simulink model "MMS_ESC_K_B_self_driving"  (R2019b)
settings: Solver=ode45  StartTime=par.sym.TStart  StopTime=par.sym.TStop  MaxStep=par.sym.max_dt  RelTol=1e-3  EnableMultiTasking=on
undefined symbols (not defined in the file): b, B_0, BASE, eta_B, eta_K, k, K_0, lambda_B, lambda_K, m, m1_B0, m1_K0, m2_B0, m2_K0, N_delay, par, Q1_B0, Q1_K0, Q2_B0, Q2_K0, sigma, T_tran, w_L, w_wav
libraries: simulink x1
settings Model: Creator=Vitù  LastModifiedBy=User
settings DataIOCC: SaveFormat=Array  SaveOutput=off  SignalLogging=off  DSMLogging=off  ReturnWorkspaceOutputs=off  TimeSaveName=TIME  OutputSaveName=Yout  OutputOption=SpecifiedOutputTimes  OutputTimes=[par.sym.TStart:par.sym.Outputdt:par.sym.TStop]
settings OptimizationCC: ExpressionDepthLimit=2147483647  LifeSpan=inf
settings DebuggingCC: UnderspecifiedInitializationDetection=Classic  MergeDetectMultiDrivingBlocksExec=none  SolverPrmCheckMsg=warning  AllowSymbolicDim=off  StateNameClashWarn=warning  SFUnexpectedBacktrackingDiag=warning  SFNoUnconditionalDefaultTransitionDiag=warning  SFExecutionAtInitializationDiag=none  ArithmeticOperatorsInVariantConditions=warning
settings HardwareCC: ProdBitPerPointer=32  ProdBitPerSizeT=32  ProdBitPerPtrDiffT=32  ProdLargestAtomicFloat=None  ProdIntDivRoundTo=Undefined  ProdEndianess=Unspecified  ProdWordSize=32  ProdHWDeviceType=32-bit Generic
settings ModelReferenceCC: PropagateSignalLabelsOutOfModel=off
settings SFSimCC: SimUseLocalCustomCode=off  CustomCodeUndefinedFunction=UseInterfaceOnly
settings RTWCC: RTWUseLocalCustomCode=off
settings CodeAppCC: StateflowObjectComments=on
settings GRTTargetCC: TargetLangStandard=C89/C90 (ANSI)  GeneratePreprocessorConditionals=Disable all
settings ConfigComp: CovMetricSettings=dw  CovHtmlReporting=on  CovSaveCumulativeToWorkspaceVar=on  CovSaveSingleToWorkspaceVar=on  CovExternalEMLEnable=off  CovSFcnEnable=off
settings SimscapeCC: SimscapeNormalizeSystem=off
settings ConfigurationSet: Description=SimMechanics 2G

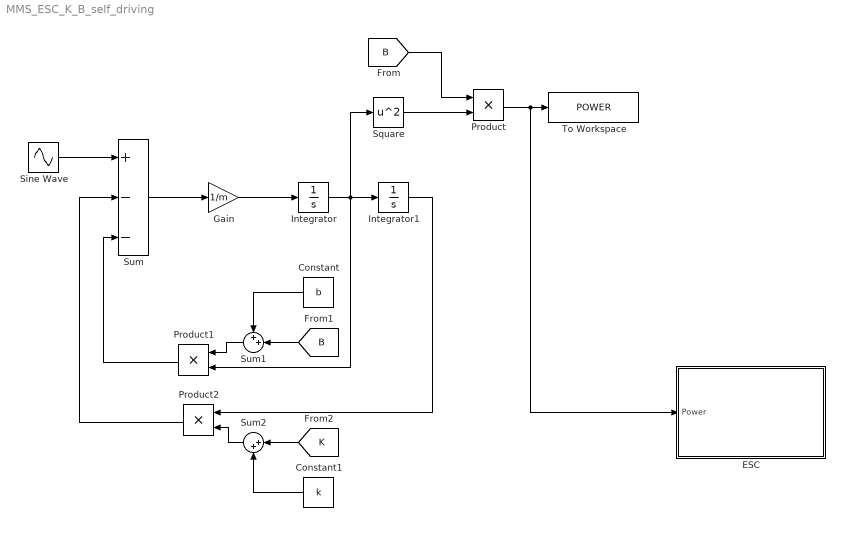
== system MMS_ESC_K_B_self_driving ==
  Constant : Constant  Value=b
  Constant1 : Constant  Value=k
  ESC : Subsystem
  Gain : Gain  Gain=1/m
  Integrator : Integrator
  Integrator1 : Integrator
  Product : Product
  Product1 : Product
  Product2 : Product
  Sine Wave : Sin  Amplitude=par.H  Frequency=w_wav  SampleTime=0
  Square : Math  Operator=square  SignedPower=off  SaturateOnIntegerOverflow=on
  Sum : Sum  Inputs=+--
  Sum1 : Sum  Inputs=++|
  Sum2 : Sum  Inputs=|++
  To Workspace : ToWorkspace  VariableName=POWER  SampleTime=-1
  wires:
  Integrator1/1 -> Product2/1
  Product/1 -> ESC/1(Power), To Workspace/1
  Product1/1 -> Sum/3
  Gain/1 -> Integrator/1
  Square/1 -> Product/2
  Sum/1 -> Gain/1
  Integrator/1 -> Product1/2, Square/1, Integrator1/1
  Product2/1 -> Sum/2
  Sine Wave/1 -> Sum/1
  [B] -> Product/1
  [B] -> Sum1/2
  Sum1/1 -> Product1/1
  Constant/1 -> Sum1/1
  [K] -> Sum2/1
  Sum2/1 -> Product2/2
  Constant1/1 -> Sum2/2

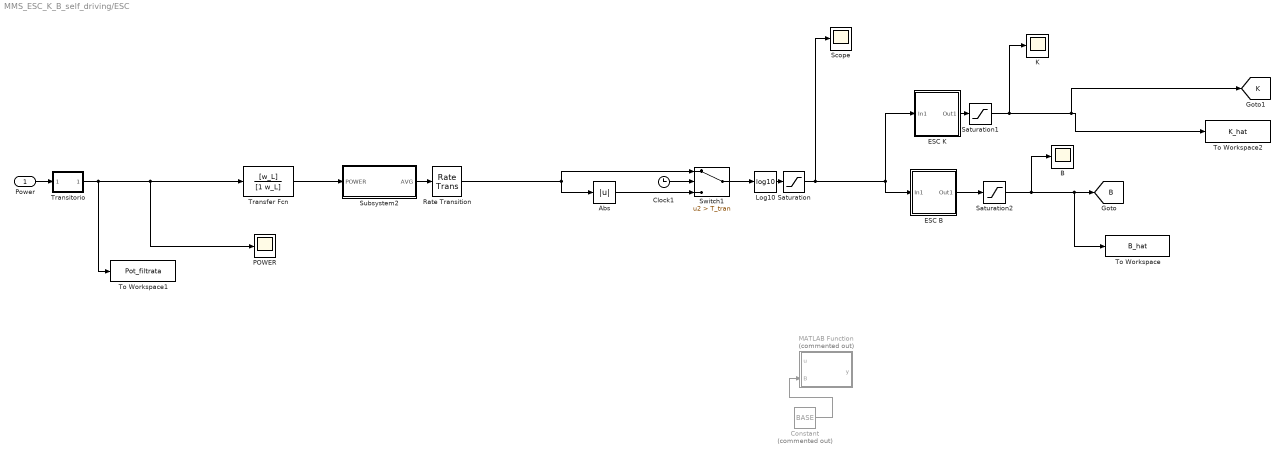
== system MMS_ESC_K_B_self_driving/ESC ==
  Power : Inport
  Abs : Abs
  B : Scope
  Clock1 : Clock
  Constant : Constant  Commented=on  Value=BASE
  ESC B : Subsystem
  ESC K : Subsystem
  K : Scope
  Log10 : Math  Operator=log10  SignedPower=off  SaturateOnIntegerOverflow=on
  MATLAB Function : MATLAB Function  Commented=on  TreatAsAtomicUnit=on
  POWER : Scope
  Rate Transition : RateTransition
  Saturation : Saturate  UpperLimit=inf  LowerLimit=-20
  Saturation1 : Saturate  UpperLimit=inf  LowerLimit=-k
  Saturation2 : Saturate  UpperLimit=inf  LowerLimit=-b
  Scope : Scope
  Subsystem2 : Subsystem
  Switch1 : Switch  Criteria=u2 > Threshold  Threshold=T_tran
  To Workspace : ToWorkspace  VariableName=B_hat  SampleTime=-1
  To Workspace1 : ToWorkspace  VariableName=Pot_filtrata  SampleTime=-1
  To Workspace2 : ToWorkspace  VariableName=K_hat  SampleTime=-1
  Transfer Fcn : TransferFcn  Numerator=[w_L]  Denominator=[1 w_L]
  Transitorio : Subsystem
  tag scope: B=global, K=global
  wires:
  Power/1 -> Transitorio/1(In1)
  ESC B/1(Out1) -> Saturation2/1
  ESC K/1(Out1) -> Saturation1/1
  Subsystem2/1(AVG) -> Rate Transition/1
  Constant/1 -> MATLAB Function/2(B)
  Log10/1 -> Saturation/1
  Transitorio/1(Out1) -> Transfer Fcn/1, POWER/1, To Workspace1/1
  Saturation/1 -> ESC B/1(In1), ESC K/1(In1), Scope/1
  Transfer Fcn/1 -> Subsystem2/1(POWER)
  Saturation1/1 -> K/1, [K], To Workspace2/1
  Saturation2/1 -> B/1, [B], To Workspace/1
  Switch1/1 -> Log10/1
  Rate Transition/1 -> Switch1/1, Abs/1
  Clock1/1 -> Switch1/2
  Abs/1 -> Switch1/3

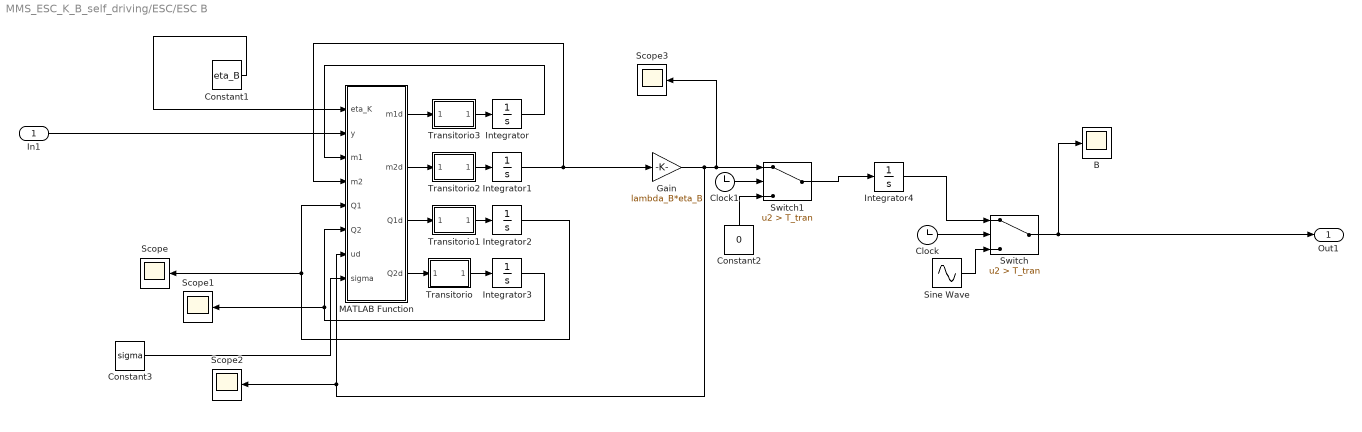
== system MMS_ESC_K_B_self_driving/ESC/ESC B ==
  In1 : Inport
  B : Scope
  Clock : Clock
  Clock1 : Clock
  Constant1 : Constant  Value=eta_B
  Constant2 : Constant  Value=0
  Constant3 : Constant  Value=sigma
  Gain : Gain  Gain=lambda_B*eta_B
  Integrator : Integrator  InitialCondition=m1_B0
  Integrator1 : Integrator  InitialCondition=m2_B0
  Integrator2 : Integrator  InitialCondition=Q1_B0
  Integrator3 : Integrator  InitialCondition=Q2_B0
  Integrator4 : Integrator  InitialCondition=B_0
  MATLAB Function : MATLAB Function  TreatAsAtomicUnit=on
  Scope{,1..3} (4 alike) : Scope
  Sine Wave : Sin  Bias=B_0  SampleTime=0
  Switch : Switch  Criteria=u2 > Threshold  Threshold=T_tran
  Switch1 : Switch  Criteria=u2 > Threshold  Threshold=T_tran
  Transitorio : Subsystem
  Transitorio1 : Subsystem
  Transitorio2 : Subsystem
  Transitorio3 : Subsystem
  Out1 : Outport
  wires:
  Switch/1 -> Out1/1, B/1
  Integrator2/1 -> MATLAB Function/5(Q1), Scope/1
  Constant2/1 -> Switch1/3
  Gain/1 -> Scope3/1, Switch1/1, MATLAB Function/7(ud), Scope2/1
  Integrator1/1 -> Gain/1, MATLAB Function/4(m2)
  MATLAB Function/4(Q2d) -> Transitorio/1(In1)
  Integrator/1 -> MATLAB Function/3(m1)
  In1/1 -> MATLAB Function/2(y)
  Switch1/1 -> Integrator4/1
  MATLAB Function/1(m1d) -> Transitorio3/1(In1)
  Integrator3/1 -> MATLAB Function/6(Q2), Scope1/1
  Sine Wave/1 -> Switch/3
  MATLAB Function/2(m2d) -> Transitorio2/1(In1)
  Clock1/1 -> Switch1/2
  MATLAB Function/3(Q1d) -> Transitorio1/1(In1)
  Constant1/1 -> MATLAB Function/1(eta_K)
  Constant3/1 -> MATLAB Function/8(sigma)
  Integrator4/1 -> Switch/1
  Clock/1 -> Switch/2
  Transitorio/1(Out1) -> Integrator3/1
  Transitorio1/1(Out1) -> Integrator2/1
  Transitorio2/1(Out1) -> Integrator1/1
  Transitorio3/1(Out1) -> Integrator/1

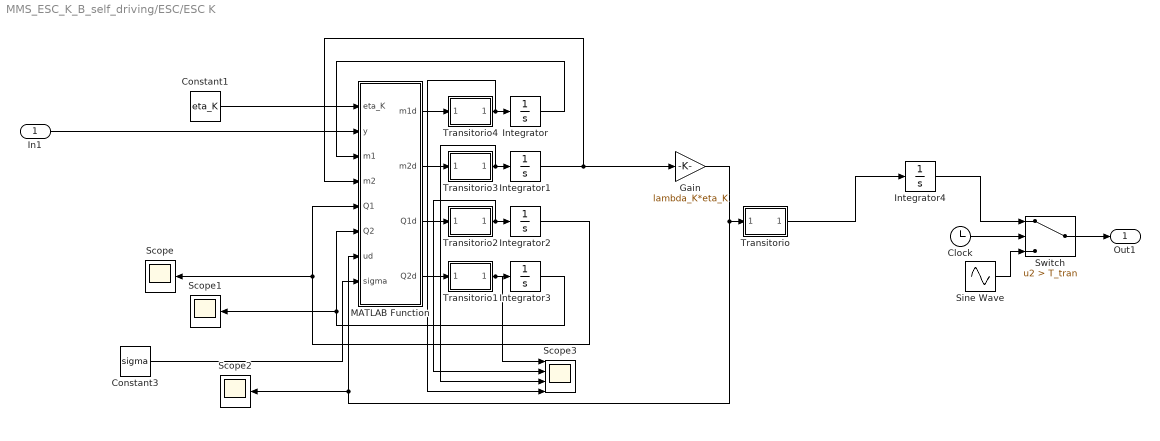
== system MMS_ESC_K_B_self_driving/ESC/ESC K ==
  In1 : Inport
  Clock : Clock
  Constant1 : Constant  Value=eta_K
  Constant3 : Constant  Value=sigma
  Gain : Gain  Gain=lambda_K*eta_K
  Integrator : Integrator  InitialCondition=m1_K0
  Integrator1 : Integrator  InitialCondition=m2_K0
  Integrator2 : Integrator  InitialCondition=Q1_K0
  Integrator3 : Integrator  InitialCondition=Q2_K0
  Integrator4 : Integrator  InitialCondition=K_0
  MATLAB Function : MATLAB Function  TreatAsAtomicUnit=on
  Scope : Scope
  Scope1 : Scope
  Scope2 : Scope
  Scope3 : Scope  NumInputPorts=4
  Sine Wave : Sin  Bias=K_0  SampleTime=0
  Switch : Switch  Criteria=u2 > Threshold  Threshold=T_tran
  Transitorio : Subsystem
  Transitorio1 : Subsystem
  Transitorio2 : Subsystem
  Transitorio3 : Subsystem
  Transitorio4 : Subsystem
  Out1 : Outport
  wires:
  Sine Wave/1 -> Switch/3
  Gain/1 -> Transitorio/1(In1), MATLAB Function/7(ud), Scope2/1
  Constant1/1 -> MATLAB Function/1(eta_K)
  Integrator1/1 -> Gain/1, MATLAB Function/4(m2)
  Integrator3/1 -> MATLAB Function/6(Q2), Scope1/1
  Integrator4/1 -> Switch/1
  Constant3/1 -> MATLAB Function/8(sigma)
  MATLAB Function/1(m1d) -> Transitorio4/1(In1)
  MATLAB Function/2(m2d) -> Transitorio3/1(In1)
  MATLAB Function/3(Q1d) -> Transitorio2/1(In1)
  Integrator/1 -> MATLAB Function/3(m1)
  MATLAB Function/4(Q2d) -> Transitorio1/1(In1)
  Clock/1 -> Switch/2
  Integrator2/1 -> MATLAB Function/5(Q1), Scope/1
  Switch/1 -> Out1/1
  In1/1 -> MATLAB Function/2(y)
  Transitorio/1(Out1) -> Integrator4/1
  Transitorio1/1(Out1) -> Scope3/1, Integrator3/1
  Transitorio2/1(Out1) -> Scope3/2, Integrator2/1
  Transitorio3/1(Out1) -> Scope3/3, Integrator1/1
  Transitorio4/1(Out1) -> Scope3/4, Integrator/1

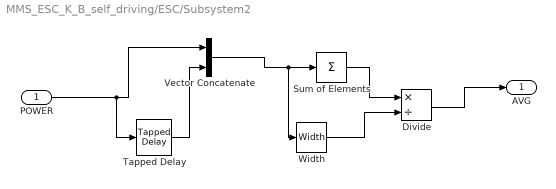
== system MMS_ESC_K_B_self_driving/ESC/Subsystem2 ==
  POWER : Inport
  Divide : Product  Inputs=*/
  Sum of Elements : Sum  Inputs=+
  Tapped Delay : simulink/Discrete/Tapped Delay  vinit=0  samptime=-1  NumDelays=N_delay  DelayOrder=Oldest  includeCurrent=off
  Vector Concatenate : Concatenate
  Width : Width
  AVG : Outport
  wires:
  POWER/1 -> Tapped Delay/1, Vector Concatenate/1
  Tapped Delay/1 -> Vector Concatenate/2
  Vector Concatenate/1 -> Width/1, Sum of Elements/1
  Sum of Elements/1 -> Divide/1
  Width/1 -> Divide/2
  Divide/1 -> AVG/1

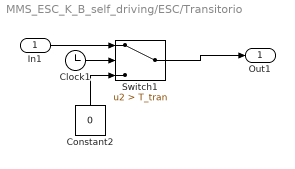
== system MMS_ESC_K_B_self_driving/ESC/Transitorio ==
  In1 : Inport
  Clock1 : Clock
  Constant2 : Constant  Value=0
  Switch1 : Switch  Criteria=u2 > Threshold  Threshold=T_tran
  Out1 : Outport
  wires:
  Constant2/1 -> Switch1/3
  Switch1/1 -> Out1/1
  Clock1/1 -> Switch1/2
  In1/1 -> Switch1/1

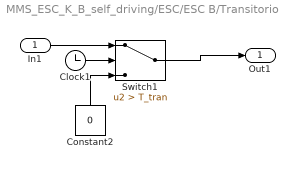
== system MMS_ESC_K_B_self_driving/ESC/ESC B/Transitorio ==
  In1 : Inport
  Clock1 : Clock
  Constant2 : Constant  Value=0
  Switch1 : Switch  Criteria=u2 > Threshold  Threshold=T_tran
  Out1 : Outport
  wires:
  Constant2/1 -> Switch1/3
  Switch1/1 -> Out1/1
  Clock1/1 -> Switch1/2
  In1/1 -> Switch1/1

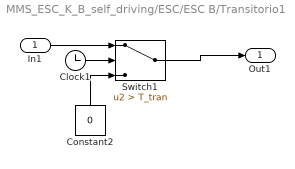
== system MMS_ESC_K_B_self_driving/ESC/ESC B/Transitorio1 ==
  In1 : Inport
  Clock1 : Clock
  Constant2 : Constant  Value=0
  Switch1 : Switch  Criteria=u2 > Threshold  Threshold=T_tran
  Out1 : Outport
  wires:
  Constant2/1 -> Switch1/3
  Switch1/1 -> Out1/1
  Clock1/1 -> Switch1/2
  In1/1 -> Switch1/1

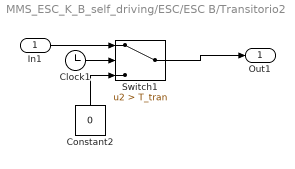
== system MMS_ESC_K_B_self_driving/ESC/ESC B/Transitorio2 ==
  In1 : Inport
  Clock1 : Clock
  Constant2 : Constant  Value=0
  Switch1 : Switch  Criteria=u2 > Threshold  Threshold=T_tran
  Out1 : Outport
  wires:
  Constant2/1 -> Switch1/3
  Switch1/1 -> Out1/1
  Clock1/1 -> Switch1/2
  In1/1 -> Switch1/1

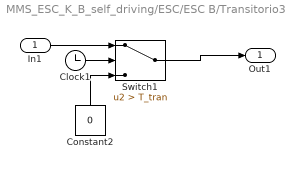
== system MMS_ESC_K_B_self_driving/ESC/ESC B/Transitorio3 ==
  In1 : Inport
  Clock1 : Clock
  Constant2 : Constant  Value=0
  Switch1 : Switch  Criteria=u2 > Threshold  Threshold=T_tran
  Out1 : Outport
  wires:
  Constant2/1 -> Switch1/3
  Switch1/1 -> Out1/1
  Clock1/1 -> Switch1/2
  In1/1 -> Switch1/1

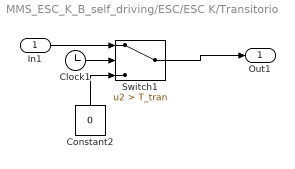
== system MMS_ESC_K_B_self_driving/ESC/ESC K/Transitorio ==
  In1 : Inport
  Clock1 : Clock
  Constant2 : Constant  Value=0
  Switch1 : Switch  Criteria=u2 > Threshold  Threshold=T_tran
  Out1 : Outport
  wires:
  Constant2/1 -> Switch1/3
  Switch1/1 -> Out1/1
  Clock1/1 -> Switch1/2
  In1/1 -> Switch1/1

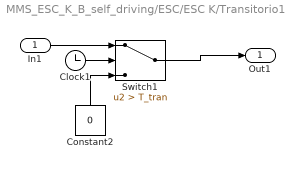
== system MMS_ESC_K_B_self_driving/ESC/ESC K/Transitorio1 ==
  In1 : Inport
  Clock1 : Clock
  Constant2 : Constant  Value=0
  Switch1 : Switch  Criteria=u2 > Threshold  Threshold=T_tran
  Out1 : Outport
  wires:
  Constant2/1 -> Switch1/3
  Switch1/1 -> Out1/1
  Clock1/1 -> Switch1/2
  In1/1 -> Switch1/1

== system MMS_ESC_K_B_self_driving/ESC/ESC K/Transitorio2 ==
  In1 : Inport
  Clock1 : Clock
  Constant2 : Constant  Value=0
  Switch1 : Switch  Criteria=u2 > Threshold  Threshold=T_tran
  Out1 : Outport
  wires:
  Constant2/1 -> Switch1/3
  Switch1/1 -> Out1/1
  Clock1/1 -> Switch1/2
  In1/1 -> Switch1/1

== system MMS_ESC_K_B_self_driving/ESC/ESC K/Transitorio3 ==
  In1 : Inport
  Clock1 : Clock
  Constant2 : Constant  Value=0
  Switch1 : Switch  Criteria=u2 > Threshold  Threshold=T_tran
  Out1 : Outport
  wires:
  Constant2/1 -> Switch1/3
  Switch1/1 -> Out1/1
  Clock1/1 -> Switch1/2
  In1/1 -> Switch1/1

== system MMS_ESC_K_B_self_driving/ESC/ESC K/Transitorio4 ==
  In1 : Inport
  Clock1 : Clock
  Constant2 : Constant  Value=0
  Switch1 : Switch  Criteria=u2 > Threshold  Threshold=T_tran
  Out1 : Outport
  wires:
  Constant2/1 -> Switch1/3
  Switch1/1 -> Out1/1
  Clock1/1 -> Switch1/2
  In1/1 -> Switch1/1

== matlab function MMS_ESC_K_B_self_driving/ESC/ESC K/MATLAB Function ==
  data: eta_K input; m1d output; y input; m1 input; m2 input; Q1 input; Q2 input; ud input; m2d output; Q1d output; Q2d output; sigma input
function [m1d,m2d,Q1d,Q2d] = SDK(eta_K,y,m1,m2,Q1,Q2,ud,sigma)
m1d = eta_K*(y-m1);
m2d = eta_K*Q1*Q2*(y-m1-Q1*m2)-sigma*eta_K*Q2*m2;
Q1d = -eta_K*Q1 + ud;
Q2d = eta_K*Q2 -eta_K*(Q1*Q2)^2-sigma*eta_K*Q2^2;

== matlab function MMS_ESC_K_B_self_driving/ESC/ESC B/MATLAB Function ==
  data: eta_K input; m1d output; y input; m1 input; m2 input; Q1 input; Q2 input; ud input; m2d output; Q1d output; Q2d output; sigma input
function [m1d,m2d,Q1d,Q2d] = SDK(eta_K,y,m1,m2,Q1,Q2,ud,sigma)
m1d = eta_K*(y-m1);
m2d = eta_K*Q1*Q2*(y-m1-Q1*m2)-sigma*eta_K*Q2*m2;
Q1d = -eta_K*Q1 + ud;
Q2d = eta_K*Q2 -eta_K*(Q1*Q2)^2-sigma*eta_K*Q2^2;

== matlab function MMS_ESC_K_B_self_driving/ESC/MATLAB Function ==
  data: u input; y output; B input
function y = fcn(u,B)
L = log(u)/log(B);
y=min([-20 L]);

y = u;
